simulink model "b_DebitMoteur"  (R2024b)
settings: Solver=FixedStepDiscrete  StartTime=0.0  StopTime=SimuPumpStop  FixedStep=0.1  RelTol=1e-6  EnableMultiTasking=on
values from neighbouring files (symbols this model uses):
  nv_remp = [0.090 0.110 0.120 0.110 0.130 0.150 0.135 0.155 0.140 0.145 0.140 0.135 0.120 0.120 ... (first row only)    [InitISM_AII.m]
  Pamb = 101300    [InitISM_AII.m]
  Rair = 287.0    (= 287)    [InitISM_AII.m]
  Tamb = 300    [InitISM_AII.m]
  Vcyl = 1998e-6/4    (= 0.0004995)    [InitISM_AII.m]
undefined symbols (not defined in the file or in its folder): PcolTest, PumpedTest, RegimeTest, TempsTest, TimePumpedTest
settings Model: Creator=a030141  LastModifiedBy=ramse
settings SolverCC: AlgebraicLoopSolver=TrustRegion
settings DataIOCC: LimitDataPoints=on  SaveFormat=Array  SignalLoggingSaveFormat=ModelDataLogs  ReturnWorkspaceOutputs=off  SignalLoggingName=sigsOut
settings OptimizationCC: InitFltsAndDblsToZero=on  LifeSpan=inf
settings DebuggingCC: SaveWithParameterizedLinksMsg=none  UnderspecifiedInitializationDetection=Classic  MergeDetectMultiDrivingBlocksExec=none  SignalResolutionControl=TryResolveAllWithWarning  MultiTaskDSMMsg=warning  MultiTaskCondExecSysMsg=none  FcnCallInpInsideContextMsg=warning  UnconnectedInputMsg=warning  UnconnectedOutputMsg=warning  UnconnectedLineMsg=warning  SFUnexpectedBacktrackingDiag=warning  SFNoUnconditionalDefaultTransitionDiag=warning  SFExecutionAtInitializationDiag=none  ArithmeticOperatorsInVariantConditions=warning
settings HardwareCC: ProdBitPerPointer=32  ProdBitPerSizeT=32  ProdBitPerPtrDiffT=32  ProdLargestAtomicFloat=None  ProdIntDivRoundTo=Undefined  ProdEndianess=Unspecified  ProdWordSize=32  ProdHWDeviceType=32-bit Generic  TargetUnknown=on
settings ModelReferenceCC: PropagateSignalLabelsOutOfModel=off
settings RTWCC: GPUComputeCapability=3.5
settings CodeAppCC: StateflowObjectComments=on
settings GRTTargetCC: TargetFcnLib=ansi_tfl_tmw.mat  TargetLangStandard=C89/C90 (ANSI)  CombineOutputUpdateFcns=off  GRTInterface=on
settings ConfigComp: CovMetricSettings=dw  CovSaveCumulativeToWorkspaceVar=on  CovSaveSingleToWorkspaceVar=on

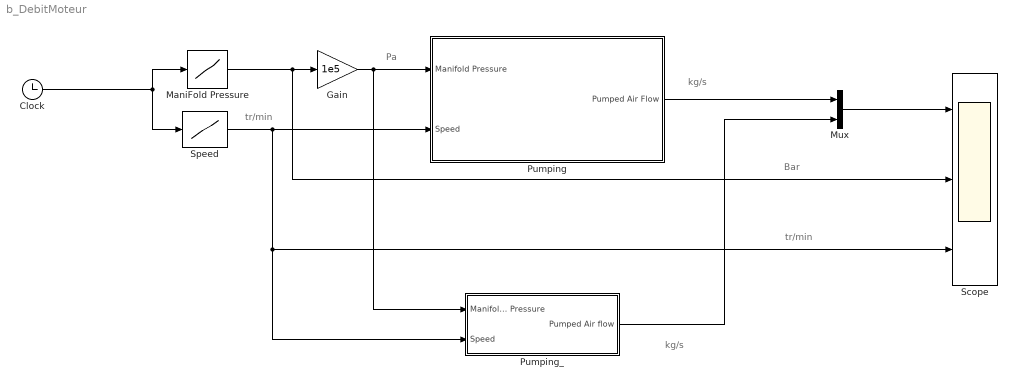
== system b_DebitMoteur ==
  note: kg/s
  note: Pa
  note: Bar
  note: tr/min
  note: tr/min
  note: kg/s
  Clock : Clock
  Gain : Gain  Gain=1e5  SaturateOnIntegerOverflow=on  OutDataTypeStr=Inherit: Same as input  ParamDataTypeStr=Inherit: Same as input
  ManiFold Pressure : Lookup  InputValues=TempsTest  Table=PcolTest
  Mux : Mux  Inputs=2
  Pumping : Subsystem
  Pumping_ : Subsystem
  Scope : Scope  NumInputPorts=3
  Speed : Lookup  InputValues=TempsTest  Table=RegimeTest
  wires:
  Speed/1 -> Pumping_/2(Speed), Scope/3, Pumping/2(Speed)
  Clock/1 -> ManiFold Pressure/1, Speed/1
  ManiFold Pressure/1 -> Gain/1, Scope/2
  Gain/1 -> Pumping_/1(Manifold Pressure), Pumping/1(Manifold Pressure)
  Mux/1 -> Scope/1
  Pumping/1(Pumped Air Flow) -> Mux/1
  Pumping_/1(Pumped Air flow) -> Mux/2

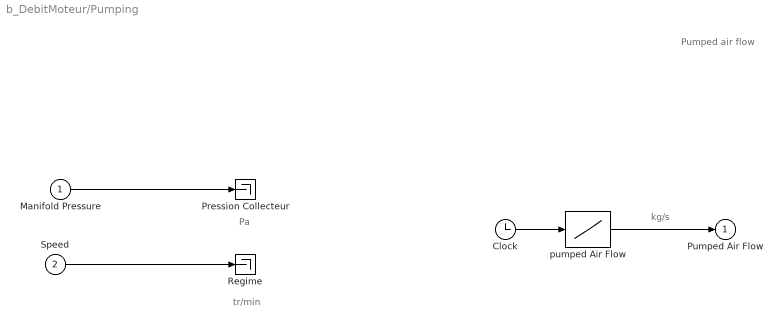
== system b_DebitMoteur/Pumping ==
  note: Pumped air flow
  note: kg/s
  note: Pa
  note: tr/min
  Manifold Pressure : Inport
  Speed : Inport  Port=2
  Clock : Clock
  Pression Collecteur : Terminator
  Regime : Terminator
  pumped Air Flow : Lookup  InputValues=TimePumpedTest  Table=PumpedTest
  Pumped Air Flow : Outport
  wires:
  Manifold Pressure/1 -> Pression Collecteur/1
  Speed/1 -> Regime/1
  pumped Air Flow/1 -> Pumped Air Flow/1
  Clock/1 -> pumped Air Flow/1

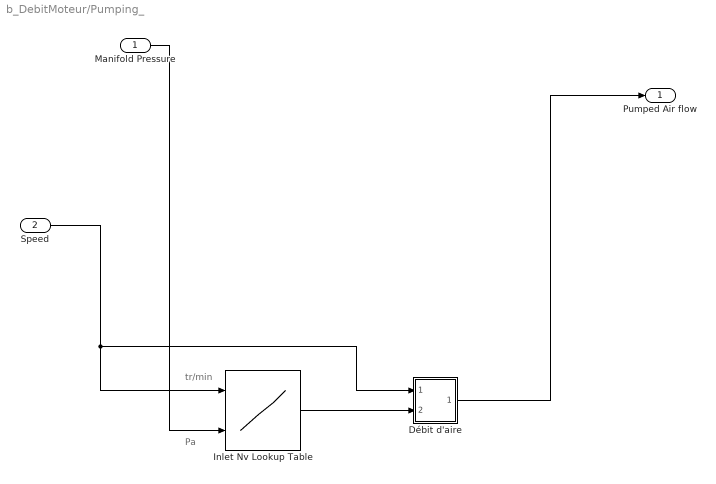
== system b_DebitMoteur/Pumping_ ==
  note: Pa
  note: tr/min
  Manifold Pressure : Inport
  Speed : Inport  Port=2
  Débit d'aire : Subsystem
  Inlet Nv Lookup Table : Lookup2D  RowIndex=Ne_remp  ColumnIndex=Pcol_remp  Table=nv_remp
  Pumped Air flow : Outport
  wires:
  Inlet Nv Lookup Table/1 -> Débit d'aire/2(In2)
  Speed/1 -> Inlet Nv Lookup Table/1, Débit d'aire/1(In1)
  Manifold Pressure/1 -> Inlet Nv Lookup Table/2
  Débit d'aire/1(Out1) -> Pumped Air flow/1

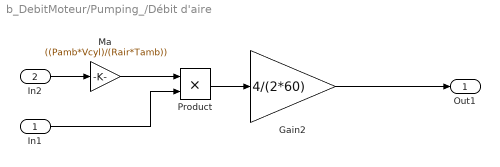
== system b_DebitMoteur/Pumping_/Débit d'aire ==
  In1 : Inport
  In2 : Inport  Port=2
  Gain2 : Gain  Gain=4/(2*60)
  Ma : Gain  Gain=((Pamb*Vcyl)/(Rair*Tamb))
  Product : Product
  Out1 : Outport
  wires:
  Ma/1 -> Product/1
  Gain2/1 -> Out1/1
  Product/1 -> Gain2/1
  In1/1 -> Product/2
  In2/1 -> Ma/1
